simulink model "vlbi_complex_dsp_core"  (Simulink 7.0)
settings: Solver=ode45  StartTime=0.0  StopTime=400  RelTol=1e-3
undefined symbols (not defined in the file or in its folder): pfb_coeff_gen_calc
libraries: xbsIndex_r4 x981, casper_library_misc x40, casper_library_delays x38, simulink x7, vlbi_lib x4, casper_library_reorder x2, casper_library_ffts_twiddle x1
(part 1 of 13)
settings Model: Creator=mdexter  LastModifiedBy=mdexter

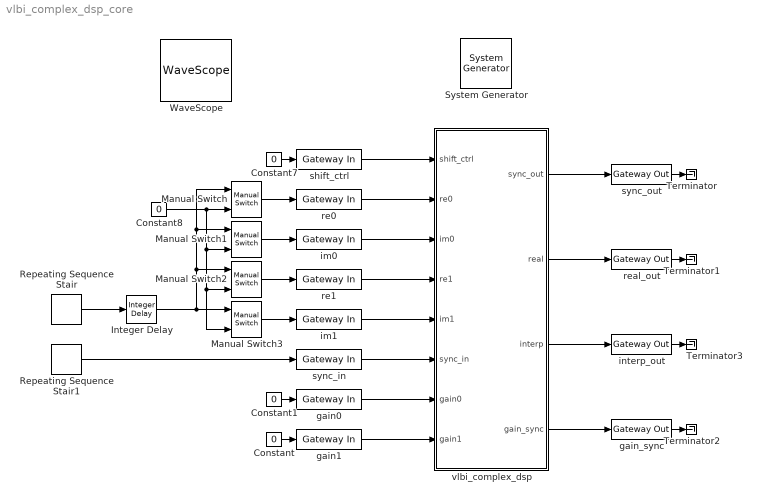
== system vlbi_complex_dsp_core ==
  " System Generator" : xbsIndex_r4/ System Generator  Tag=genX  SystemSampleTime=-1  xilinxfamily=virtex2p  part=xc2vp50  speed=-7  package=ff1152  synthesis_tool=XST  clock_wrapper=Clock Enables  directory=./vlbi_complex_dsp_core  testbench=off  simulink_period=1  sysclk_period=100  dcm_input_clock_period=100  incr_netlist=off  trim_vbits=Everywhere in SubSystem  dbl_ovrd=According to Block Masks  core_generation=According to Block Masks  run_coregen=off  deprecated_control=off  eval_field=0  block_type=sysgen
      settings: block_version=10.1.3
  Constant{,1,7..8} (4 alike) : Constant  Value=0
  Integer Delay : simulink/Discrete/Integer Delay  vinit=0.0  samptime=1  NumDelays=1
  Manual Switch : simulink/Signal Routing/Manual Switch  SystemSampleTime=-1  sw=1  action=0  varsize=off
  Manual Switch1 : simulink/Signal Routing/Manual Switch  SystemSampleTime=-1  sw=0  action=0  varsize=off
  Manual Switch2 : simulink/Signal Routing/Manual Switch  SystemSampleTime=-1  sw=1  action=0  varsize=off
  Manual Switch3 : simulink/Signal Routing/Manual Switch  SystemSampleTime=-1  sw=0  action=0  varsize=off
  Repeating Sequence Stair : simulink/Sources/Repeating Sequence Stair  SystemSampleTime=-1  OutValues=[1 zeros(1,7)]*0.5  tsamp=1  OutMin=[]  OutMax=[]  OutDataTypeStr=float('double')  OutputDataTypeScalingMode=Specify via dialog  OutDataType=float('double')  ConRadixGroup=Best Precision: Vector-wise  OutScaling=2^-12
  Repeating Sequence Stair1 : simulink/Sources/Repeating Sequence Stair  SystemSampleTime=-1  OutValues=[1, zeros(1,32-1)]  tsamp=1  OutMin=[]  OutMax=[]  OutDataTypeStr=float('double')  OutputDataTypeScalingMode=Specify via dialog  OutDataType=float('double')  ConRadixGroup=Best Precision: Vector-wise  OutScaling=2^-12
  Terminator{,1..3} (4 alike) : Terminator
  WaveScope : xbsIndex_r4/WaveScope  block_type=wavescope
      settings: block_version=10.1.3
  gain0 : xbsIndex_r4/Gateway In  arith_type="Signed  (2's comp)"  n_bits=32  bin_pt=0  quantization="Round  (unbiased: +/- Inf)"  overflow=Saturate  period=1  dbl_ovrd=off  timing_constraint=None  locs_specified=off  LOCs={}  block_type=gatewayin
      settings: infoedit="Gateway in block.  Converts inputs of type Simulink integer, double and fixed point to  Xilinx fixed point type.<P><P>Hardware notes:  In hardware these blocks become top level input ports."  block_version=10.1.3
  gain1 : xbsIndex_r4/Gateway In  arith_type="Signed  (2's comp)"  n_bits=32  bin_pt=0  quantization="Round  (unbiased: +/- Inf)"  overflow=Saturate  period=1  dbl_ovrd=off  timing_constraint=None  locs_specified=off  LOCs={}  block_type=gatewayin
      settings: infoedit="Gateway in block.  Converts inputs of type Simulink integer, double and fixed point to  Xilinx fixed point type.<P><P>Hardware notes:  In hardware these blocks become top level input ports."  block_version=10.1.3
  gain_sync : xbsIndex_r4/Gateway Out  hdl_port=on  timing_constraint=None  locs_specified=off  LOCs={}  block_type=gatewayout
      settings: infoedit="Gateway out block.  Converts Xilinx fixed point inputs into ouputs of type Simulink integer, double, or fixed point.<P><P>Hardware notes:  In hardware these blocks become top level output ports or are discarded, depending on how they are configured."  block_version=10.1.3
  im0 : xbsIndex_r4/Gateway In  arith_type="Signed  (2's comp)"  n_bits=8  bin_pt=7  quantization="Round  (unbiased: +/- Inf)"  overflow=Saturate  period=1  dbl_ovrd=off  timing_constraint=None  locs_specified=off  LOCs={}  block_type=gatewayin
      settings: infoedit="Gateway in block.  Converts inputs of type Simulink integer, double and fixed point to  Xilinx fixed point type.<P><P>Hardware notes:  In hardware these blocks become top level input ports."  block_version=10.1.3
  im1 : xbsIndex_r4/Gateway In  arith_type="Signed  (2's comp)"  n_bits=8  bin_pt=7  quantization="Round  (unbiased: +/- Inf)"  overflow=Saturate  period=1  dbl_ovrd=off  timing_constraint=None  locs_specified=off  LOCs={}  block_type=gatewayin
      settings: infoedit="Gateway in block.  Converts inputs of type Simulink integer, double and fixed point to  Xilinx fixed point type.<P><P>Hardware notes:  In hardware these blocks become top level input ports."  block_version=10.1.3
  interp_out : xbsIndex_r4/Gateway Out  hdl_port=on  timing_constraint=None  locs_specified=off  LOCs={}  block_type=gatewayout
      settings: infoedit="Gateway out block.  Converts Xilinx fixed point inputs into ouputs of type Simulink integer, double, or fixed point.<P><P>Hardware notes:  In hardware these blocks become top level output ports or are discarded, depending on how they are configured."  block_version=10.1.3
  re0 : xbsIndex_r4/Gateway In  arith_type="Signed  (2's comp)"  n_bits=8  bin_pt=7  quantization="Round  (unbiased: +/- Inf)"  overflow=Saturate  period=1  dbl_ovrd=off  timing_constraint=None  locs_specified=off  LOCs={}  block_type=gatewayin
      settings: infoedit="Gateway in block.  Converts inputs of type Simulink integer, double and fixed point to  Xilinx fixed point type.<P><P>Hardware notes:  In hardware these blocks become top level input ports."  block_version=10.1.3
  re1 : xbsIndex_r4/Gateway In  arith_type="Signed  (2's comp)"  n_bits=8  bin_pt=7  quantization="Round  (unbiased: +/- Inf)"  overflow=Saturate  period=1  dbl_ovrd=off  timing_constraint=None  locs_specified=off  LOCs={}  block_type=gatewayin
      settings: infoedit="Gateway in block.  Converts inputs of type Simulink integer, double and fixed point to  Xilinx fixed point type.<P><P>Hardware notes:  In hardware these blocks become top level input ports."  block_version=10.1.3
  real_out : xbsIndex_r4/Gateway Out  hdl_port=on  timing_constraint=None  locs_specified=off  LOCs={}  block_type=gatewayout
      settings: infoedit="Gateway out block.  Converts Xilinx fixed point inputs into ouputs of type Simulink integer, double, or fixed point.<P><P>Hardware notes:  In hardware these blocks become top level output ports or are discarded, depending on how they are configured."  block_version=10.1.3
  shift_ctrl : xbsIndex_r4/Gateway In  arith_type=Unsigned  n_bits=32  bin_pt=0  quantization="Round  (unbiased: +/- Inf)"  overflow=Saturate  period=1  dbl_ovrd=off  timing_constraint=None  locs_specified=off  LOCs={}  block_type=gatewayin
      settings: infoedit="Gateway in block.  Converts inputs of type Simulink integer, double and fixed point to  Xilinx fixed point type.<P><P>Hardware notes:  In hardware these blocks become top level input ports."  block_version=10.1.3
  sync_in : xbsIndex_r4/Gateway In  arith_type=Boolean  n_bits=16  bin_pt=14  quantization="Round  (unbiased: +/- Inf)"  overflow=Saturate  period=1  dbl_ovrd=off  timing_constraint=None  locs_specified=off  LOCs={}  block_type=gatewayin
      settings: infoedit="Gateway in block.  Converts inputs of type Simulink integer, double and fixed point to  Xilinx fixed point type.<P><P>Hardware notes:  In hardware these blocks become top level input ports."  block_version=10.1.3
  sync_out : xbsIndex_r4/Gateway Out  hdl_port=on  timing_constraint=None  locs_specified=off  LOCs={}  block_type=gatewayout
      settings: infoedit="Gateway out block.  Converts Xilinx fixed point inputs into ouputs of type Simulink integer, double, or fixed point.<P><P>Hardware notes:  In hardware these blocks become top level output ports or are discarded, depending on how they are configured."  block_version=10.1.3
  vlbi_complex_dsp : Subsystem
  wires:
  Constant/1 -> gain1/1
  Constant1/1 -> gain0/1
  Constant7/1 -> shift_ctrl/1
  shift_ctrl/1 -> vlbi_complex_dsp/1(shift_ctrl)
  re0/1 -> vlbi_complex_dsp/2(re0)
  im0/1 -> vlbi_complex_dsp/3(im0)
  re1/1 -> vlbi_complex_dsp/4(re1)
  im1/1 -> vlbi_complex_dsp/5(im1)
  sync_in/1 -> vlbi_complex_dsp/6(sync_in)
  gain0/1 -> vlbi_complex_dsp/7(gain0)
  gain1/1 -> vlbi_complex_dsp/8(gain1)
  sync_out/1 -> Terminator/1
  real_out/1 -> Terminator1/1
  gain_sync/1 -> Terminator2/1
  interp_out/1 -> Terminator3/1
  vlbi_complex_dsp/1(sync_out) -> sync_out/1
  vlbi_complex_dsp/2(real) -> real_out/1
  vlbi_complex_dsp/3(interp) -> interp_out/1
  vlbi_complex_dsp/4(gain_sync) -> gain_sync/1
  Repeating Sequence Stair/1 -> Integer Delay/1
  Integer Delay/1 -> Manual Switch3/1, Manual Switch2/1, Manual Switch/1, Manual Switch1/1
  Constant8/1 -> Manual Switch/2, Manual Switch1/2, Manual Switch3/2, Manual Switch2/2
  Repeating Sequence Stair1/1 -> sync_in/1
  Manual Switch3/1 -> im1/1
  Manual Switch2/1 -> re1/1
  Manual Switch1/1 -> im0/1
  Manual Switch/1 -> re0/1

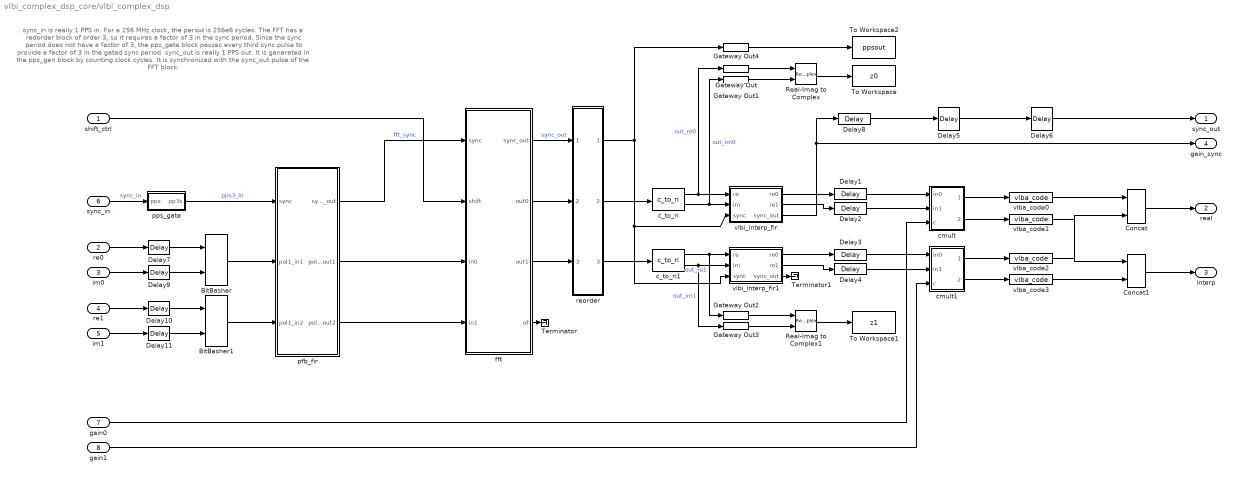
== system vlbi_complex_dsp_core/vlbi_complex_dsp ==
  note: sync_in is really 1 PPS in.  For a 256 MHz clock, the period is 256e6 cycles.
      | The FFT has a redorder block of order 3, so it requires a factor of 3 in the sync
      | period.  Since the sync period does not have a factor of 3, the pps_gate block
      | passes every third sync pulse to provide a factor of 3 in the gated sync period.
      |
      | sync_out is really 1 PPS out.  It is generated in the pps_gen block by counting
      | clock cycles.  It is synchronized with the sync_out pulse of the FFT block.
  shift_ctrl : Inport  OutDataType=sfix(16)  OutScaling=2^0
  re0 : Inport  Port=2  OutDataType=sfix(16)  OutScaling=2^0
  im0 : Inport  Port=3  OutDataType=sfix(16)  OutScaling=2^0
  re1 : Inport  Port=4  OutDataType=sfix(16)  OutScaling=2^0
  im1 : Inport  Port=5  OutDataType=sfix(16)  OutScaling=2^0
  sync_in : Inport  Port=6  OutDataType=sfix(16)  OutScaling=2^0
  gain0 : Inport  Port=7  OutDataType=sfix(16)  OutScaling=2^0
  gain1 : Inport  Port=8  OutDataType=sfix(16)  OutScaling=2^0
  BitBasher : xbsIndex_r4/BitBasher  bitexpr=|  display_expr=off  sr_1=1  arith_type1=Unsigned  bin_pt1=0  sr_2=2  arith_type2=Unsigned  bin_pt2=0  sr_3=3  arith_type3=Unsigned  bin_pt3=0  sr_4=4  arith_type4=Unsigned  bin_pt4=0  dbl_ovrd=off  block_type=bitbasher
      | <html><head><meta name="qrichtext" content="1" /><style type="text/css">
      | p, li { white-space: pre-wrap; }
      | </style></head><body style=" font-family:'MS Shell Dlg 2'; font-size:8.25pt; font-weight:400; font-style:normal;">
      | <p style=" margin-top:12px; margin-bottom:12px; margin-left:0px; margin-right:0px; -qt-block-indent:0; text-indent:0px; font-family:'MS Shell Dlg'; font-size:8pt;">a_bi={a,b}</p></body></html>
      settings: block_version=10.1.3
  BitBasher1 : xbsIndex_r4/BitBasher  bitexpr=|  display_expr=off  sr_1=1  arith_type1=Unsigned  bin_pt1=0  sr_2=2  arith_type2=Unsigned  bin_pt2=0  sr_3=3  arith_type3=Unsigned  bin_pt3=0  sr_4=4  arith_type4=Unsigned  bin_pt4=0  dbl_ovrd=off  block_type=bitbasher
      | <html><head><meta name="qrichtext" content="1" /><style type="text/css">
      | p, li { white-space: pre-wrap; }
      | </style></head><body style=" font-family:'MS Shell Dlg 2'; font-size:8.25pt; font-weight:400; font-style:normal;">
      | <p style=" margin-top:12px; margin-bottom:12px; margin-left:0px; margin-right:0px; -qt-block-indent:0; text-indent:0px; font-family:'MS Shell Dlg'; font-size:8pt;">a_bi={a,b}</p></body></html>
      settings: block_version=10.1.3
  Concat : xbsIndex_r4/Concat  num_inputs=2  dbl_ovrd=off  block_type=concat
      settings: block_version=11.3
  Concat1 : xbsIndex_r4/Concat  num_inputs=2  dbl_ovrd=off  block_type=concat
      settings: block_version=11.3
  Delay1 : xbsIndex_r4/Delay  en=off  latency=1  dbl_ovrd=off  reg_retiming=off  block_type=delay
      settings: xl_area=[0, 0, 0, 0, 0, 0, 0]  block_version=11.3
  Delay{7,9..11} (4 alike) : xbsIndex_r4/Delay  en=off  latency=2  dbl_ovrd=off  reg_retiming=off  block_type=delay
      settings: xl_area=[0, 0, 0, 0, 0, 0, 0]  block_version=11.3
  Delay{2..4,8} (4 alike) : xbsIndex_r4/Delay  en=off  latency=1  dbl_ovrd=off  reg_retiming=on  block_type=delay
      settings: xl_area=[0, 0, 0, 0, 0, 0, 0]  block_version=11.3
  Delay5 : xbsIndex_r4/Delay  en=off  latency=5  dbl_ovrd=off  reg_retiming=off  block_type=delay
      settings: xl_area=[0, 0, 0, 0, 0, 0, 0]  block_version=11.3
  Delay6 : xbsIndex_r4/Delay  en=off  latency=6  dbl_ovrd=off  reg_retiming=off  block_type=delay
      settings: xl_area=[0, 0, 0, 0, 0, 0, 0]  block_version=11.3
  Gateway Out{,1..4} (5 alike) : xbsIndex_r4/Gateway Out  hdl_port=off  timing_constraint=None  locs_specified=off  LOCs={}  block_type=gatewayout
      settings: infoedit="Gateway out block.  Converts Xilinx fixed point inputs into ouputs of type Simulink integer, double, or fixed point.<P><P>Hardware notes:  In hardware these blocks become top level output ports or are discarded, depending on how they are configured."  block_version=10.1.3
  Real-Imag to Complex : RealImagToComplex
  Real-Imag to Complex1 : RealImagToComplex
  Terminator : Terminator
  Terminator1 : Terminator
  To Workspace : ToWorkspace  VariableName=z0  SampleTime=-1  SaveFormat=Array
  To Workspace1 : ToWorkspace  VariableName=z1  SampleTime=-1  SaveFormat=Array
  To Workspace2 : ToWorkspace  VariableName=ppsout  SampleTime=-1  SaveFormat=Array
  c_to_ri : casper_library_misc/c_to_ri  SystemSampleTime=-1  n_bits=18  bin_pt=17
  c_to_ri1 : casper_library_misc/c_to_ri  SystemSampleTime=-1  n_bits=18  bin_pt=17
  cmult : Subsystem  mask{n_bits=18, mult_latency=3}
      mask prompts: n_bits "Bit Width"; mult_latency "Mult Latency"
  cmult1 : Subsystem  mask{n_bits=18, mult_latency=3}
      mask prompts: n_bits "Bit Width"; mult_latency "Mult Latency"
  fft : Subsystem  AncestorBlock=casper_library_ffts/fft  mask(fft){FFTSize=4, n_inputs=1, input_bit_width=18, coeff_bit_width=18, unscramble=on, add_latency=2, mult_latency=3, bram_latency=2, conv_latency=2, quantization=Round  (unbiased: Even Values), overflow=Saturate, arch=Virtex2Pro, opt_target=logic, coeffs_bit_limit=8, delays_bit_limit=9, specify_mult=off, mult_spec=, hardcode_shifts=off, shift_schedule=, dsp48_adders=off}
      mask prompts: FFTSize "Size of FFT: (2^? pts)"; n_inputs "Number of Simultaneous Inputs: (2^?)"; input_bit_width "Input/Output Bit Width"; coeff_bit_width "Coefficient Bit Width"; unscramble "Unscramble output (ie, put channels in canonical order)"; add_latency "Add Latency"; mult_latency "Mult Latency"; bram_latency "BRAM Latency"; conv_latency "Convert Latency"; quantization "Quantization Behavior"; overflow "Overflow Behavior"; arch "Architecture"; opt_target "Use less"; coeffs_bit_limit "Number bits above which to store stage's coefficients in BRAM (2^? bits)"; delays_bit_limit "Number bits above which to store stage's delays in BRAM (2^? bits)"; specify_mult "Specify multiplier use (behavioral HDL if not specified)"; mult_spec "Multiplier specification (0=core, 1=embedded, 2=behavioural) (left=1st stage)"; hardcode_shifts "Hardcode shift schedule"; shift_schedule "Shift schedule"; dsp48_adders "DSP48 adders in butterfly"
      mask help: A complex FFT.
      mask init:
      | fft_init(gcb, ...
      |     'FFTSize', FFTSize, ...
      |     'n_inputs', n_inputs, ...
      |     'input_bit_width', input_bit_width, ...
      |     'coeff_bit_width', coeff_bit_width, ...
      |     'unscramble', unscramble, ...
      |     'add_latency', add_latency, ...
      |     'mult_latency', mult_latency, ...
      |     'bram_latency', bram_latency, ...
      |     'conv_latency', conv_latency, ...
      |     'quantization', quantization, ...
      |     'overflow', overflow, ...
      |     'arch', arch, ...
      |     'opt_target', opt_target, ...
      |     'coeffs_bit_limit', coeffs_bit_limit, ...
      |     'delays_bit_limit', delays_bit_limit, ...
      |     'specify_mult', specify_mult, ...
      |     'mult_spec', mult_spec, ...
      |     'hardcode_shifts', hardcode_shifts, ...
      |     'shift_schedule', shift_schedule, ...
      |     'dsp48_adders', dsp48_adders);
      settings: CopyFcn=fft_init(gcb);
      settings: AttributesFormatString=|
      | 4 stages
      | (18,18)
      | Round  (unbiased: Even Values)
      | Saturate
      mask Help: eval('xlWeb(''http://casper.berkeley.edu/wiki/Fft'')')
      mask StyleString: edit,edit,edit,edit,checkbox,edit,edit,edit,edit,popup(Truncate|Round  (unbiased: +/- Inf)|Round  (unbiased: Even Values)),popup(Wrap|Saturate|Error),popup(Virtex2Pro|Virtex5),popup(logic|multipliers),edit,edit,checkbox,edit,checkbox,edit,checkbox
      mask CallbackString:
      | |||||||||||fft_callback_arch(gcb);||||specify_mult = get_param(gcb, 'specify_mult');
      | set_param_state(gcb, 'mult_spec', specify_mult);||hardcode_shifts = get_param(gcb, 'hardcode_shifts');
      | set_param_state(gcb, 'shift_schedule', hardcode_shifts);||fft_callback_dsp48_adders(gcb);
      mask TabNameString: Basic,Basic,Basic,Basic,Basic,Latency,Latency,Latency,Latency,Implementation,Implementation,Implementation,Implementation,Implementation,Implementation,Implementation,Implementation,Implementation,Implementation,Implementation
  pfb_fir : Subsystem  AncestorBlock=casper_library_pfbs/pfb_fir  mask(pfb_fir){PFBSize=4, TotalTaps=8, WindowType=hamming, n_inputs=1, MakeBiplex=0, BitWidthIn=8, BitWidthOut=18, CoeffBitWidth=8, CoeffDistMem=0, add_latency=2, mult_latency=3, bram_latency=2, quantization=Round  (unbiased: Even Values), fwidth=1, specify_mult=off, mult_spec=[2                                      2]}
      mask prompts: PFBSize "Size of PFB: (2^? pnts)"; TotalTaps "Total Number of Taps:"; WindowType "Windowing Function:"; n_inputs "Number of Simultaneous Inputs: (2^?)"; MakeBiplex "Make Biplex"; BitWidthIn "Input Bitwidth:"; BitWidthOut "Output Bitwidth:"; CoeffBitWidth "Coefficient Bitwidth:"; CoeffDistMem "Use Distributed Memory for Coeffs"; add_latency "Add Latency"; mult_latency "Mult Latency"; bram_latency "BRAM Latency"; quantization "Quantization Behavior"; fwidth "Bin Width Scaling (normal=1)"; specify_mult "Specify multiplier use (behavioral if not specified)"; mult_spec "Multiplier specification (0=core, 1=embedded, 2=behavioural) (left=1st tap)"
      mask init:
      | pfb_fir_init(gcb, ...
      |     'PFBSize', PFBSize, ...
      |     'TotalTaps', TotalTaps, ...
      |     'WindowType', WindowType, ...
      |     'n_inputs', n_inputs, ...
      |     'MakeBiplex', MakeBiplex, ...
      |     'BitWidthIn', BitWidthIn, ...
      |     'BitWidthOut', BitWidthOut, ...
      |     'CoeffBitWidth', CoeffBitWidth, ...
      |     'CoeffDistMem', CoeffDistMem, ...
      |     'add_latency', add_latency, ...
      |     'mult_latency', mult_latency, ...
      |     'bram_latency', bram_latency, ...
      |     'quantization', quantization, ...
      |     'fwidth', fwidth,...
      |     'specify_mult', specify_mult,...
      |     'mult_spec', mult_spec);
      settings: AttributesFormatString=|
      | taps=8, add_latency=2
      | max scale 0.821
      mask Help: eval('xlWeb(''http://casper.berkeley.edu/wiki/Pfb_fir'')')
      mask StyleString: edit,edit,popup(bartlett|barthannwin|blackman|blackmanharris|bohamwin|chebwin|flattopwin|gausswin|hamming|hann|kaiser|nuttallwin|parzenwin|rectwin|tukeywin|triang|userwindow),edit,edit,edit,edit,edit,edit,edit,edit,edit,popup(Truncate|Round  (unbiased: +/- Inf)|Round  (unbiased: Even Values)),edit,checkbox,edit
      mask CallbackString:
      | |%num_taps = eval(get_param(gcb, 'TotalTaps'));
      | %old_vec = eval(get_param(gcb, 'mult_spec'));
      | 
      | %vec = 2.*ones(1,num_taps);
      | %old_size = length(old_vec);
      | 
      | %if(old_size <= num_taps),
      | %   new_size = old_size;
      | %else,
      | %    new_size = num_taps;
      | %end
      | 
      | %for n = 1:new_size, vec(n) = old_vec(n); end
      | %set_param(gcb, 'mult_spec', mat2str(vec));||||||||||||%num_taps = eval(get_param(gcb, 'TotalTaps'));
      | %old_vec = eval(get_param(gcb, 'mult_spec'));
      | 
      | %vec = 2.*ones(1,num_taps);
      | %old_size = length(old_vec);
      | 
      | %if(old_size <= num_taps),
      | %    new_size = old_size;
      | %else,
      | %    new_size = num_taps;
      | %end
      | 
      | %for n = 1:new_size, vec(n) = old_vec(n); end
      | %set_param(gcb, 'mult_spec', mat2str(vec));|%specify_mult = get_param(gcb,'specify_mult');
      | %if( strcmp(specify_mult,'off')),
      | %    set_param(gcb, 'MaskEnables', {'on','on','on','on','on','on','on','on','on','on','on','on','on','on','on','off'});
      | %else
      | %    set_param(gcb, 'MaskEnables', {'on','on','on','on','on','on','on','on','on','on','on','on','on','on','on','on'});
      | %end
      | 
      | |%specify_mult = get_param(gcb,'specify_mult');
      | %if( strcmp(specify_mult,'off')),
      | %    set_param(gcb, 'MaskEnables', {'on','on','on','on','on','on','on','on','on','on','on','on','on','on','on','off'});
      | %else
      | %    set_param(gcb, 'MaskEnables', {'on','on','on','on','on','on','on','on','on','on','on','on','on','on','on','on'});
      | %end
  pps_gate : Subsystem
  reorder : Subsystem
  vlba_code{0..3} (4 alike) : vlbi_lib/vlba_code  SystemSampleTime=-1  bitwidth=18
  vlbi_interp_fir : Subsystem  mask{tap_delay=8, n_bits=18, add_latency=3, mult_latency=4, bram_latency=2}
      mask prompts: tap_delay "Delay between Taps"; n_bits "Bit Width"; add_latency "Add Latency"; mult_latency "Mult Latency"; bram_latency "BRAM Latency"
      mask init:
      | for i=0:4,
      |     x = pi*(2*i+1)/2;
      |     coeff(i+1) = sin(x)/x;
      | end
      | coeff = coeff / (2*sum(coeff));
  vlbi_interp_fir1 : Subsystem  mask{tap_delay=8, n_bits=18, add_latency=3, mult_latency=4, bram_latency=2}
      mask prompts: tap_delay "Delay between Taps"; n_bits "Bit Width"; add_latency "Add Latency"; mult_latency "Mult Latency"; bram_latency "BRAM Latency"
      mask init:
      | for i=0:4,
      |     x = pi*(2*i+1)/2;
      |     coeff(i+1) = sin(x)/x;
      | end
      | coeff = coeff / (2*sum(coeff));
  sync_out : Outport  OutDataType=sfix(16)  OutScaling=2^0
  real : Outport  Port=2
  interp : Outport  Port=3
  gain_sync : Outport  Port=4  OutDataType=sfix(16)  OutScaling=2^0
  wires:
  sync_in/1 -> pps_gate/1(pps)  "sync_in"
  re0/1 -> Delay7/1
  re1/1 -> Delay10/1
  im1/1 -> Delay11/1
  c_to_ri/1 -> vlbi_interp_fir/1(re), Gateway Out/1  "out_re0"
  c_to_ri/2 -> vlbi_interp_fir/2(im), Gateway Out1/1  "out_im0"
  c_to_ri1/1 -> vlbi_interp_fir1/1(re), Gateway Out2/1  "out_re1"
  c_to_ri1/2 -> vlbi_interp_fir1/2(im), Gateway Out3/1  "out_im1"
  vlbi_interp_fir/1(re0) -> Delay1/1
  vlbi_interp_fir/2(re1) -> Delay2/1
  vlbi_interp_fir1/1(re0) -> Delay3/1
  vlbi_interp_fir1/2(re1) -> Delay4/1
  vlbi_interp_fir/3(sync_out) -> Delay8/1, gain_sync/1
  Delay6/1 -> sync_out/1
  vlba_code0/1 -> Concat/1
  vlba_code1/1 -> Concat1/1
  vlba_code2/1 -> Concat/2
  vlba_code3/1 -> Concat1/2
  im0/1 -> Delay9/1
  shift_ctrl/1 -> fft/2(shift)
  Delay8/1 -> Delay5/1
  Delay5/1 -> Delay6/1
  Delay1/1 -> cmult/1(in0)
  Delay2/1 -> cmult/2(in1)
  Delay3/1 -> cmult1/1(in0)
  Delay4/1 -> cmult1/2(in1)
  gain0/1 -> cmult/3(c)
  gain1/1 -> cmult1/3(c)
  cmult/1(out0) -> vlba_code0/1
  cmult/2(out1) -> vlba_code1/1
  cmult1/1(out0) -> vlba_code2/1
  cmult1/2(out1) -> vlba_code3/1
  fft/3(out1) -> reorder/3(in1)
  pps_gate/1(pp3s) -> pfb_fir/1(sync)  "pps3_in"
  pfb_fir/1(sync_out) -> fft/1(sync)  "fft_sync"
  fft/1(sync_out) -> reorder/1(pp3s)  "sync_out"
  fft/2(out0) -> reorder/2(in0)
  fft/4(of) -> Terminator/1
  vlbi_interp_fir1/3(sync_out) -> Terminator1/1
  Concat/1 -> real/1
  Concat1/1 -> interp/1
  reorder/1(pps) -> vlbi_interp_fir/3(sync), vlbi_interp_fir1/3(sync), Gateway Out4/1
  reorder/2(out0) -> c_to_ri/1
  reorder/3(out1) -> c_to_ri1/1
  BitBasher/1 -> pfb_fir/2(pol1_in1)
  Delay7/1 -> BitBasher/1
  Delay9/1 -> BitBasher/2
  BitBasher1/1 -> pfb_fir/3(pol1_in2)
  Delay10/1 -> BitBasher1/1
  Delay11/1 -> BitBasher1/2
  pfb_fir/2(pol1_out1) -> fft/3(in0)
  pfb_fir/3(pol1_out2) -> fft/4(in1)
  Real-Imag to Complex/1 -> To Workspace/1
  Gateway Out/1 -> Real-Imag to Complex/1
  Gateway Out1/1 -> Real-Imag to Complex/2
  Real-Imag to Complex1/1 -> To Workspace1/1
  Gateway Out2/1 -> Real-Imag to Complex1/1
  Gateway Out3/1 -> Real-Imag to Complex1/2
  Gateway Out4/1 -> To Workspace2/1

== system vlbi_complex_dsp_core/vlbi_complex_dsp/cmult ==
  in0 : Inport  OutDataType=sfix(16)  OutScaling=2^0
  in1 : Inport  Port=2  OutDataType=sfix(16)  OutScaling=2^0
  c : Inport  Port=3  OutDataType=sfix(16)  OutScaling=2^0
  Convert : xbsIndex_r4/Convert  arith_type="Signed  (2's comp)"  n_bits=n_bits  bin_pt=n_bits-1  quantization=Truncate  overflow=Saturate  latency=2  dbl_ovrd=off  pipeline=on  block_type=convert
      settings: xl_area=[0, 0, 0, 0, 0, 0, 0]  block_version=11.3
  Convert1 : xbsIndex_r4/Convert  arith_type="Signed  (2's comp)"  n_bits=n_bits  bin_pt=n_bits-1  quantization=Truncate  overflow=Saturate  latency=2  dbl_ovrd=off  pipeline=on  block_type=convert
      settings: xl_area=[0, 0, 0, 0, 0, 0, 0]  block_version=11.3
  Delay8 : xbsIndex_r4/Delay  en=off  latency=2  dbl_ovrd=off  reg_retiming=on  block_type=delay
      settings: xl_area=[0, 0, 0, 0, 0, 0, 0]  block_version=11.3
  Reinterpret : xbsIndex_r4/Reinterpret  force_arith_type=on  arith_type=Unsigned  force_bin_pt=on  bin_pt=6  block_type=reinterpret
      settings: infoedit="Changes signal type without altering the binary representation.   You can changed the signal between signed and unsigned, and relocate the binary point.<br><br>Hardware notes: In hardware this block costs nothing.<br><br>Example:  Suppose the input is 6 bits wide, signed, with 2 fractional bits, and the output is forced to unsigned with 0 fractional bits.  Then an input of -2.0 (1110.00 in binary 2's complement) becomes an output of 56 (111000 in binary)."  block_version=11.3
  Slice : xbsIndex_r4/Slice  nbits=n_bits  boolean_output=off  mode=Lower Bit Location + Width  bit1=0  base1=MSB of Input  bit0=0  base0=LSB of Input  dbl_ovrd=off  block_type=slice
      settings: block_version=11.3
  ac : xbsIndex_r4/Mult  precision=Full  arith_type="Signed  (2's comp)"  n_bits=8  bin_pt=2  quantization=Truncate  overflow=Wrap  en=off  latency=mult_latency  dbl_ovrd=off  use_behavioral_HDL=off  use_embedded=on  opt=Speed  optimum_pipeline=off  pipeline=on  use_rpm=on  placement_style=Rectangular shape  block_type=mult
      settings: xl_area=[0, 0, 0, 0, 0, 0, 0]  block_version=11.3
  bd : xbsIndex_r4/Mult  precision=Full  arith_type="Signed  (2's comp)"  n_bits=8  bin_pt=2  quantization=Truncate  overflow=Wrap  en=off  latency=mult_latency  dbl_ovrd=off  use_behavioral_HDL=off  use_embedded=on  opt=Speed  optimum_pipeline=off  pipeline=on  use_rpm=on  placement_style=Rectangular shape  block_type=mult
      settings: xl_area=[0, 0, 0, 0, 0, 0, 0]  block_version=11.3
  out0 : Outport  OutDataType=sfix(16)  OutScaling=2^0
  out1 : Outport  Port=2  OutDataType=sfix(16)  OutScaling=2^0
  wires:
  Slice/1 -> Delay8/1
  in0/1 -> Convert/1
  in1/1 -> Convert1/1
  ac/1 -> out0/1
  bd/1 -> out1/1
  Reinterpret/1 -> bd/2, ac/2
  c/1 -> Slice/1
  Convert/1 -> ac/1
  Convert1/1 -> bd/1
  Delay8/1 -> Reinterpret/1

== system vlbi_complex_dsp_core/vlbi_complex_dsp/cmult1 ==
  in0 : Inport  OutDataType=sfix(16)  OutScaling=2^0
  in1 : Inport  Port=2  OutDataType=sfix(16)  OutScaling=2^0
  c : Inport  Port=3  OutDataType=sfix(16)  OutScaling=2^0
  Convert : xbsIndex_r4/Convert  arith_type="Signed  (2's comp)"  n_bits=n_bits  bin_pt=n_bits-1  quantization=Truncate  overflow=Saturate  latency=2  dbl_ovrd=off  pipeline=on  block_type=convert
      settings: xl_area=[0, 0, 0, 0, 0, 0, 0]  block_version=11.3
  Convert1 : xbsIndex_r4/Convert  arith_type="Signed  (2's comp)"  n_bits=n_bits  bin_pt=n_bits-1  quantization=Truncate  overflow=Saturate  latency=2  dbl_ovrd=off  pipeline=on  block_type=convert
      settings: xl_area=[0, 0, 0, 0, 0, 0, 0]  block_version=11.3
  Delay8 : xbsIndex_r4/Delay  en=off  latency=2  dbl_ovrd=off  reg_retiming=on  block_type=delay
      settings: xl_area=[0, 0, 0, 0, 0, 0, 0]  block_version=11.3
  Reinterpret : xbsIndex_r4/Reinterpret  force_arith_type=on  arith_type=Unsigned  force_bin_pt=on  bin_pt=6  block_type=reinterpret
      settings: infoedit="Changes signal type without altering the binary representation.   You can changed the signal between signed and unsigned, and relocate the binary point.<br><br>Hardware notes: In hardware this block costs nothing.<br><br>Example:  Suppose the input is 6 bits wide, signed, with 2 fractional bits, and the output is forced to unsigned with 0 fractional bits.  Then an input of -2.0 (1110.00 in binary 2's complement) becomes an output of 56 (111000 in binary)."  block_version=11.3
  Slice : xbsIndex_r4/Slice  nbits=n_bits  boolean_output=off  mode=Lower Bit Location + Width  bit1=0  base1=MSB of Input  bit0=0  base0=LSB of Input  dbl_ovrd=off  block_type=slice
      settings: block_version=11.3
  ac : xbsIndex_r4/Mult  precision=Full  arith_type="Signed  (2's comp)"  n_bits=8  bin_pt=2  quantization=Truncate  overflow=Wrap  en=off  latency=mult_latency  dbl_ovrd=off  use_behavioral_HDL=off  use_embedded=on  opt=Speed  optimum_pipeline=off  pipeline=on  use_rpm=on  placement_style=Rectangular shape  block_type=mult
      settings: xl_area=[0, 0, 0, 0, 0, 0, 0]  block_version=11.3
  bd : xbsIndex_r4/Mult  precision=Full  arith_type="Signed  (2's comp)"  n_bits=8  bin_pt=2  quantization=Truncate  overflow=Wrap  en=off  latency=mult_latency  dbl_ovrd=off  use_behavioral_HDL=off  use_embedded=on  opt=Speed  optimum_pipeline=off  pipeline=on  use_rpm=on  placement_style=Rectangular shape  block_type=mult
      settings: xl_area=[0, 0, 0, 0, 0, 0, 0]  block_version=11.3
  out0 : Outport  OutDataType=sfix(16)  OutScaling=2^0
  out1 : Outport  Port=2  OutDataType=sfix(16)  OutScaling=2^0
  wires:
  Delay8/1 -> Reinterpret/1
  Convert1/1 -> bd/1
  Convert/1 -> ac/1
  c/1 -> Slice/1
  Reinterpret/1 -> ac/2, bd/2
  bd/1 -> out1/1
  ac/1 -> out0/1
  in1/1 -> Convert1/1
  in0/1 -> Convert/1
  Slice/1 -> Delay8/1

== system vlbi_complex_dsp_core/vlbi_complex_dsp/fft ==
  sync : Inport
  shift : Inport  Port=2
  in0 : Inport  Port=3
  in1 : Inport  Port=4
  fft_biplex0 : Subsystem  AncestorBlock=casper_library_ffts/fft_biplex  mask(fft_biplex){FFTSize=3, input_bit_width=18, coeff_bit_width=18, add_latency=2, mult_latency=3, bram_latency=2, conv_latency=2, quantization=Round  (unbiased: Even Values), overflow=Saturate, arch=Virtex2Pro, opt_target=logic, coeffs_bit_limit=8, delays_bit_limit=9, specify_mult=off, mult_spec=[2                                      2                                      2], hardcode_shifts=off, shift_schedule=[1                                      1                                      1], dsp48_adders=off}
      mask prompts: FFTSize "Size of FFT: (2^? pts)"; input_bit_width "Input/Output Bit Width"; coeff_bit_width "Coefficient Bit Width"; add_latency "Add Latency"; mult_latency "Mult Latency"; bram_latency "BRAM Latency"; conv_latency "Convert latency"; quantization "Quantization Behavior"; overflow "Overflow Behavior"; arch "Architecture"; opt_target "Use less"; coeffs_bit_limit "Number bits above which to store stage's coefficients in BRAM (2^? bits)"; delays_bit_limit "Number bits above which to implent stage's delays in BRAM (2^? bits)"; specify_mult "Specify multiplier use (behavioral HDL if not specified)"; mult_spec "Multiplier specification (0=core, 1=embedded, 2=behavioural) (left=1st stage)"; hardcode_shifts "Hardcode shift schedule"; shift_schedule "Shift schedule"; dsp48_adders "Use DSP48s for adders"
      mask help: FFT internal block.
      mask init:
      | fft_biplex_init(gcb, ...
      |     'FFTSize', FFTSize, ...
      |     'input_bit_width', input_bit_width, ...
      |     'coeff_bit_width', coeff_bit_width, ...
      |     'add_latency', add_latency, ...
      |     'mult_latency', mult_latency, ...
      |     'bram_latency', bram_latency, ...
      |     'conv_latency', conv_latency, ...
      |     'quantization', quantization, ...
      |     'overflow', overflow, ...
      |     'arch', arch, ...
      |     'opt_target', opt_target, ...
      |     'coeffs_bit_limit', coeffs_bit_limit, ...
      |     'delays_bit_limit', delays_bit_limit, ...
      |     'specify_mult', specify_mult, ...
      |     'mult_spec', mult_spec, ...
      |     'hardcode_shifts', hardcode_shifts, ...
      |     'shift_schedule', shift_schedule, ...
      |     'dsp48_adders', dsp48_adders);
      settings: AttributesFormatString=|
      | 3 stages
      | Virtex2Pro
      mask StyleString: edit,edit,edit,edit,edit,edit,edit,popup(Truncate|Round  (unbiased: +/- Inf)|Round  (unbiased: Even Values)),popup(Wrap|Saturate|Error),popup(Virtex2Pro|Virtex5),popup(logic|multipliers),edit,edit,checkbox,edit,checkbox,edit,checkbox
      mask CallbackString:
      | |||||||||fft_callback_arch(gcb);||||specify_mult = get_param(gcb, 'specify_mult');
      | set_param_state(gcb, 'mult_spec', specify_mult);||hardcode_shifts = get_param(gcb, 'hardcode_shifts');
      | set_param_state(gcb, 'shift_schedule', hardcode_shifts);||fft_callback_dsp48_adders(gcb);
      mask TabNameString: Basic,Basic,Basic,Latency,Latency,Latency,Latency,Implementation,Implementation,Implementation,Implementation,Implementation,Implementation,Implementation,Implementation,Implementation,Implementation,Implementation
  fft_direct : Subsystem  AncestorBlock=casper_library_ffts/fft_direct  mask(fft_direct){FFTSize=1, input_bit_width=18, coeff_bit_width=18, map_tail=on, LargerFFTSize=4, StartStage=4, add_latency=2, mult_latency=3, bram_latency=2, conv_latency=2, quantization=Round  (unbiased: Even Values), overflow=Saturate, arch=Virtex2Pro, opt_target=logic, coeffs_bit_limit=8, specify_mult=off, mult_spec=2, hardcode_shifts=off, shift_schedule=1, dsp48_adders=off}
      mask prompts: FFTSize "Size of FFT: (2^? pts)"; input_bit_width "Input/Output Bit Width"; coeff_bit_width "Coefficient Bit Width"; map_tail "Map Tail of Larger FFT"; LargerFFTSize "Size of Larger FFT (2^?)"; StartStage "Start Stage of Map Tail"; add_latency "Add Latency"; mult_latency "Mult Latency"; bram_latency "BRAM Latency"; conv_latency "Convert latency"; quantization "Quantization Behavior"; overflow "Overflow Behavior"; arch "Architecture"; opt_target "Use less"; coeffs_bit_limit "Number bits above which to store stage's coefficients in BRAM (2^? bits)"; specify_mult "Specify multiplier use (behavioural HDL if not specified)"; mult_spec "Multiplier specification (0=core, 1=behavioural HDL, 2=embedded) (left=1st stage)"; hardcode_shifts "Hardcode shift schedule"; shift_schedule "Shift schedule"; dsp48_adders "DSP48 adders in butterfly"
      mask help:
      | FFT internal block.
      |
      | Implements an N-point FFT as the classic butterfly structure,
      | with N inputs and N outputs.
      mask init:
      | fft_direct_init(gcb, ...
      |     'FFTSize', FFTSize, ...
      |     'input_bit_width', input_bit_width, ...
      |     'coeff_bit_width', coeff_bit_width, ...
      |     'map_tail', map_tail, ...
      |     'LargerFFTSize', LargerFFTSize, ...
      |     'StartStage', StartStage, ...
      |     'add_latency', add_latency, ...
      |     'mult_latency', mult_latency, ...
      |     'bram_latency', bram_latency, ...
      |     'conv_latency', conv_latency, ...
      |     'quantization', quantization, ...
      |     'overflow', overflow, ...
      |     'arch', arch, ...
      |     'opt_target', opt_target, ...
      |     'coeffs_bit_limit', coeffs_bit_limit, ...
      |     'specify_mult', specify_mult, ...
      |     'mult_spec', mult_spec, ...
      |     'hardcode_shifts', hardcode_shifts, ...
      |     'shift_schedule', shift_schedule, ...
      |     'dsp48_adders', dsp48_adders);
      settings: AttributesFormatString=|
      | Virtex2Pro
      | stages [4] of 4
      | [18,18]
      | Round  (unbiased: Even Values)
      | Saturate
      mask StyleString: edit,edit,edit,checkbox,edit,edit,edit,edit,edit,edit,popup(Truncate|Round  (unbiased: +/- Inf)|Round  (unbiased: Even Values)),popup(Wrap|Saturate|Error),popup(Virtex2Pro|Virtex5),popup(logic|multipliers),edit,checkbox,edit,checkbox,edit,checkbox
      mask CallbackString:
      | |||map_tail = get_param(gcb, 'map_tail');
      | set_param_state(gcb, 'LargerFFTSize', map_tail);
      | set_param_state(gcb, 'StartStage', map_tail);|||||||||fft_callback_arch(gcb);|||specify_mult = get_param(gcb, 'specify_mult');
      | set_param_state(gcb, 'mult_spec', specify_mult);||hardcode_shifts = get_param(gcb, 'hardcode_shifts');
      | set_param_state(gcb, 'shift_schedule', hardcode_shifts);||fft_callback_dsp48_adders(gcb);
      mask TabNameString: Basic,Basic,Basic,Basic,Basic,Basic,Latency,Latency,Latency,Latency,Implementation,Implementation,Implementation,Implementation,Implementation,Implementation,Implementation,Implementation,Implementation,Implementation
  fft_unscrambler : Subsystem  AncestorBlock=casper_library_ffts/fft_unscrambler  mask(fft_unscrambler){FFTSize=4, n_inputs=1, bram_latency=2}
      mask prompts: FFTSize "Size of FFT: (2^?)"; n_inputs "Number of Simultaneous Inputs: (2^?)"; bram_latency "BRAM Latency"
      mask init:
      | fft_unscrambler_init(gcb,...
      |     'FFTSize',FFTSize,... 
      |     'n_inputs', n_inputs,...
      |     'bram_latency', bram_latency);
      settings: AttributesFormatString=FFTSize=4, n_inputs=1
  of_or : xbsIndex_r4/Logical  logical_function=OR  inputs=2  en=off  latency=1  precision=Full  arith_type=Unsigned  n_bits=16  bin_pt=0  align_bp=on  dbl_ovrd=off  block_type=logical
  slice : xbsIndex_r4/Slice  nbits=1  boolean_output=off  mode=Lower Bit Location + Width  bit1=0  base1=MSB of Input  bit0=3  base0=LSB of Input  dbl_ovrd=off  block_type=slice
      settings: infoedit="Extracts a given range of bits from each input sample and presents it at the output.  The output type is ordinarily unsigned with binary point at zero, but can be Boolean when the slice is one bit wide.<P><P>Hardware notes: In hardware this block costs nothing."  block_version=10.1.3
  sync_out : Outport
  out0 : Outport  Port=2
  out1 : Outport  Port=3
  of : Outport  Port=4
  wires:
  sync/1 -> fft_biplex0/1(sync)
  shift/1 -> fft_biplex0/2(shift), slice/1
  in0/1 -> fft_biplex0/3(pol1)
  in1/1 -> fft_biplex0/4(pol2)
  fft_biplex0/4(of) -> of_or/2
  slice/1 -> fft_direct/2(shift)
  fft_biplex0/1(sync_out) -> fft_direct/1(sync)
  fft_biplex0/2(pol1_out) -> fft_direct/3(in0)
  fft_biplex0/3(pol2_out) -> fft_direct/4(in1)
  fft_direct/4(of) -> of_or/1
  of_or/1 -> of/1
  fft_direct/1(sync_out) -> fft_unscrambler/1(sync)
  fft_unscrambler/1(sync_out) -> sync_out/1
  fft_direct/2(out0) -> fft_unscrambler/2(In1)
  fft_unscrambler/2(Out1) -> out0/1
  fft_direct/3(out1) -> fft_unscrambler/3(In2)
  fft_unscrambler/3(Out2) -> out1/1
